simulink model "power_mutual"  (Simulink 6.0)
settings: Solver=ode45  SolverMode=SingleTasking  StartTime=0.0  StopTime=0.1  RelTol=1e-3  AbsTol=1e-6
libraries: powerlib x8
settings Model: Creator=patrice  LastModifiedBy=batserve  ExtModeTrigMode=oneshot  ExtModeArmWhenConnect=off  ExtModeAutoUpdateStatusClock=off
settings DataIOCC: LimitDataPoints=off  SignalLoggingName=sigsOut
settings OptimizationCC: BlockReduction=off  BooleanDataType=off
settings DebuggingCC: SolverPrmCheckMsg=none
settings HardwareCC: TargetUnknown=on
settings RTWCC: TemplateMakefile=grt_unix.tmf

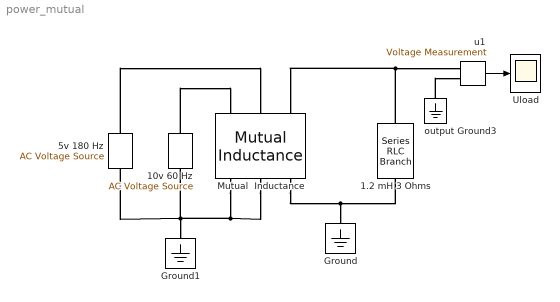
== system power_mutual ==
  1.2 mH 3 Ohms : powerlib/Elements/Series RLC Branch  Orientation=up  PhysicalDomain=powersysdomain  SubClassName=unknown  PortType=p1  LConnTagsString=__new0  RConnTagsString=__new0  Resistance=3  Inductance=1.2e-03  Capacitance=inf  Measurements=None
  10v 60 Hz : powerlib/Electrical Sources/AC Voltage Source  Description=source block  Orientation=up  Amplitude=10  Phase=0  Frequency=60  SampleTime=0  Measurements=None
      settings: AttributesFormatString=\n
  5v 180 Hz : powerlib/Electrical Sources/AC Voltage Source  Description=source block  Orientation=up  Amplitude=5  Phase=0  Frequency=180  SampleTime=0  Measurements=None
      settings: AttributesFormatString=\n
  Ground : powerlib/Elements/Ground  Orientation=down  PhysicalDomain=powersysdomain  SubClassName=unknown  PortType=p1  LConnTagsString=a
  Ground1 : powerlib/Elements/Ground  Orientation=down  PhysicalDomain=powersysdomain  SubClassName=unknown  PortType=p1  LConnTagsString=a
  Mutual  Inductance : powerlib/Elements/Mutual Inductance  Orientation=down  PhysicalDomain=powersysdomain  SubClassName=unknown  PortType=p1  LConnTagsString=a|b|c  RConnTagsString=A|B|C  SelfImpedance1=[1.1 1.1e-03]  SelfImpedance2=[ 1.1 1.1e-03]  ThreeWindings=on  SelfImpedance3=[ 1.1 1.1e-03]  MutualImpedance=[1.0 1.0e-03]  Measurements=None
      settings: AttributesFormatString=\n
  Uload : Scope
      settings: TickLabels=on  TimeRange=0.1  YMin=-10  YMax=10  DataFormat=Array
  output Ground3 : powerlib/Elements/Ground  Orientation=down  PhysicalDomain=powersysdomain  SubClassName=unknown  PortType=p1  LConnTagsString=a
  u1 : powerlib/Measurements/Voltage Measurement  Tag=PoWeRsYsTeMmEaSuReMeNt  PhasorSimulation=off  OutputType=Magnitude  PSBequivalent=0
  wires:
  u1/1 -> Uload/1
  connections:
  Mutual  Inductance/RConn3 -- Ground/LConn1 -- 1.2 mH 3 Ohms/LConn1
  1.2 mH 3 Ohms/RConn1 -- u1/LConn1 -- Mutual  Inductance/LConn3
  output Ground3/LConn1 -- u1/LConn2
  10v 60 Hz/RConn1 -- Mutual  Inductance/LConn1
  Mutual  Inductance/RConn2 -- 5v 180 Hz/LConn1 -- 10v 60 Hz/LConn1 -- Ground1/LConn1 -- Mutual  Inductance/RConn1
  5v 180 Hz/RConn1 -- Mutual  Inductance/LConn2
